simulink model "parte_1"  (R2020b)
settings: Solver=VariableStepAuto  StartTime=0.0  StopTime=4  RelTol=1e-3
values from neighbouring files (symbols this model uses):
  A_3 = [-(R1+R2)/(R1*R2*C1), 1/(R2*C1),-1/(R2*C1);0,0,-1/(R3*C2);-1/(R2*C3),1/(R2*C3),-(R2+R3)/(R2*R3*C3)]    [Lab8.m]
  B_3 = [1/(R1*C1);0;0]    [Lab8.m]
  C_3 = [0,1,0]    [Lab8.m]
  C_new = eye(3)    [Lab8.m]
  D_3 = zeros(3,1)    [Lab8.m]
undefined symbols (not defined in the file or in its folder): Klqi
settings Model: Creator=julit  LastModifiedBy=julit

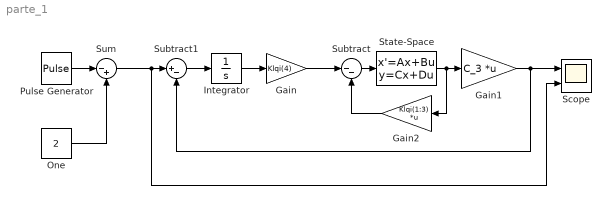
== system parte_1 ==
  Gain : Gain  Gain=Klqi(4)
  Gain1 : Gain  Gain=C_3  Multiplication=Matrix(K*u) (u vector)
  Gain2 : Gain  Gain=Klqi(1:3)  Multiplication=Matrix(K*u) (u vector)
  Integrator : Integrator
  One : Constant  Value=2  OutDataTypeStr=Inherit: Inherit via back propagation
  Pulse Generator : DiscretePulseGenerator  PulseType=Time based  PulseWidth=50
  Scope : Scope  NumInputPorts=2
  State-Space : StateSpace  A=A_3  B=B_3  C=C_new  D=D_3  InitialCondition=0
  Subtract : Sum  Inputs=|--
  Subtract1 : Sum  Inputs=|+-
  Sum : Sum  Inputs=|-+
  wires:
  Pulse Generator/1 -> Sum/1
  State-Space/1 -> Gain2/1, Gain1/1
  Subtract/1 -> State-Space/1
  Gain2/1 -> Subtract/2
  Gain/1 -> Subtract/1
  Integrator/1 -> Gain/1
  Gain1/1 -> Scope/1, Subtract1/2
  One/1 -> Sum/2
  Subtract1/1 -> Integrator/1
  Sum/1 -> Scope/2, Subtract1/1
